simulink model "radia_optuna_teaching"  (R2026a)
settings: Solver=FixedStepDiscrete  StopTime=1.4  FixedStep=0.1
model workspace (MAT data in the model file):
  radia_optuna_teaching_exercise = "quadratic"
  radia_optuna_teaching_parameters = radia.optuna.OptimizationParameter
  radia_optuna_teaching_parameters.Name = "x"
  radia_optuna_teaching_parameters.Value = 0
  radia_optuna_teaching_parameters.Minimum = -1
  radia_optuna_teaching_parameters.Maximum = 1
settings Model: Creator=Administrator  LastModifiedBy=Administrator

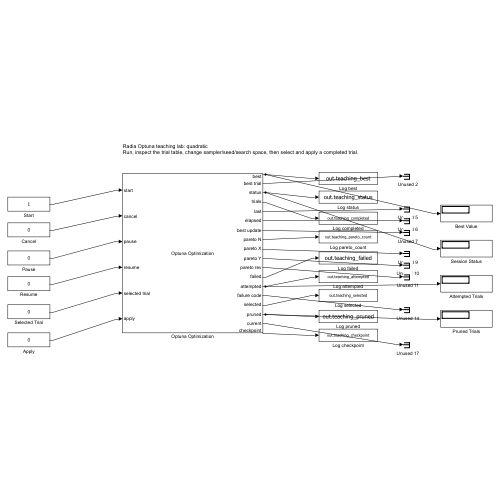
[thumbnail: Simulink's stored preview of the top-level diagram]
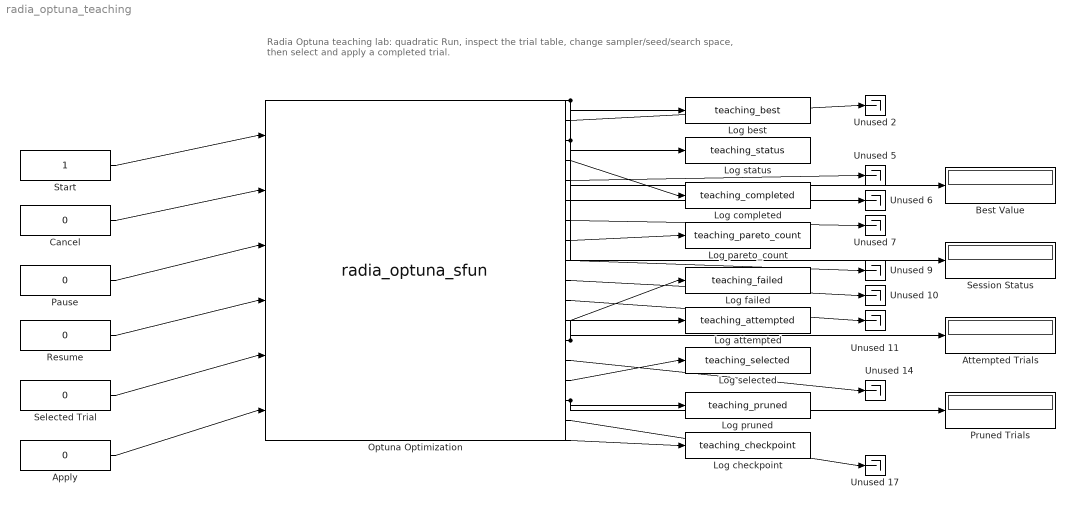
== system radia_optuna_teaching ==
  note: Radia Optuna teaching lab: quadratic
      | Run, inspect the trial table, change sampler/seed/search space, then select and apply a completed trial.
  Apply : Constant  Value=0
  Attempted Trials : Display
  Best Value : Display
  Cancel : Constant  Value=0
  Log attempted : ToWorkspace  VariableName=teaching_attempted  SampleTime=-1
  Log best : ToWorkspace  VariableName=teaching_best  SampleTime=-1
  Log checkpoint : ToWorkspace  VariableName=teaching_checkpoint  SampleTime=-1
  Log completed : ToWorkspace  VariableName=teaching_completed  SampleTime=-1
  Log failed : ToWorkspace  VariableName=teaching_failed  SampleTime=-1
  Log pareto_count : ToWorkspace  VariableName=teaching_pareto_count  SampleTime=-1
  Log pruned : ToWorkspace  VariableName=teaching_pruned  SampleTime=-1
  Log selected : ToWorkspace  VariableName=teaching_selected  SampleTime=-1
  Log status : ToWorkspace  VariableName=teaching_status  SampleTime=-1
  Optuna Optimization : M-S-Function  Description=MATLAB-native Optuna session. One trial executes per sample; completed history is checkpointed and objective failures are recorded. Status: -1 failure, 0 idle, 1 complete, 2 running, 3 cancelled, 4 paused.  FunctionName=radia_optuna_sfun  Parameters=objective_fcn,num_trials,directions,storage_path,sample_time_s,strcmp(live_visualization,'on'),struct('Name',sampler_name,'Seed',seed,'Pruner',pruner_name,'Parameters',parameter_spec,'ModelName',model_name)  mask{objective_fcn='radia.optuna.teachingQuadraticObjective', num_trials=12, directions="minimize", storage_path='C:\temp\radia_optuna_teaching_quadratic.mat', sample_time_s=0.10000000000000001, live_visualization=off, sampler_name=tpe, seed=20260829, pruner_name=median, parameter_spec=radia_optuna_teaching_parameters, model_name='radia_optuna_teaching'}
      mask prompts: objective_fcn "Objective function"; num_trials "Number of trials"; directions "Objective directions"; storage_path "Study MAT file"; sample_time_s "Trial sample time (s)"; live_visualization "External MATLAB monitor"; sampler_name "Sampler"; seed "Sampler seed ([] = fresh)"; pruner_name "Pruner"; parameter_spec "OptimizationParameter array ([] = Trial objective)"; model_name "Model to update"
      mask help: MATLAB-native Optuna session. One trial executes per sample; completed history is checkpointed and objective failures are recorded. Status: -1 failure, 0 idle, 1 complete, 2 running, 3 cancelled, 4 paused.
      mask TypeOptions sampler_name: auto | random | tpe | cmaes | motpe | nsgaii | gp | nsgaiii | bruteforce | qmc
      mask TypeOptions pruner_name: none | median | hyperband | percentile | patient | successivehalving | threshold
      mask Display: disp('Optuna Optimization');port_label('input',1,'start');port_label('input',2,'cancel');port_label('input',3,'pause');port_label('input',4,'resume');port_label('input',5,'selected trial');port_label('input',6,'apply');port_label('output',1,'best');port_label('output',2,'best trial');port_label('output',3,'status');port_label('output',4,'trials');port_label('output',5,'last');port_label('output',6,'elapsed');port_label('output',7,'best update');port_label('output',8,'pareto N');port_label('output',9,'pareto X');port_label('output',10,'pareto Y');port_label('output',11,'pareto rev');port_label('output',12,'failed');port_label('output',13,'attempted');port_label('output',14,'failure code');port_label('output',15,'selected');port_label('output',16,'pruned');port_label('output',17,'current');port_label('output',18,'checkpoint');
  Pause : Constant  Value=0
  Pruned Trials : Display
  Resume : Constant  Value=0
  Selected Trial : Constant  Value=0
  Session Status : Display
  Start : Constant
  Unused {2,5..7,9..11,14,17} (9 alike) : Terminator
  wires:
  Start/1 -> Optuna Optimization/1
  Cancel/1 -> Optuna Optimization/2
  Pause/1 -> Optuna Optimization/3
  Resume/1 -> Optuna Optimization/4
  Selected Trial/1 -> Optuna Optimization/5
  Apply/1 -> Optuna Optimization/6
  Optuna Optimization/1 -> Log best/1, Best Value/1
  Optuna Optimization/3 -> Log status/1, Session Status/1
  Optuna Optimization/4 -> Log completed/1
  Optuna Optimization/8 -> Log pareto_count/1
  Optuna Optimization/12 -> Log failed/1
  Optuna Optimization/13 -> Log attempted/1, Attempted Trials/1
  Optuna Optimization/15 -> Log selected/1
  Optuna Optimization/16 -> Log pruned/1, Pruned Trials/1
  Optuna Optimization/18 -> Log checkpoint/1
  Optuna Optimization/2 -> Unused 2/1
  Optuna Optimization/5 -> Unused 5/1
  Optuna Optimization/6 -> Unused 6/1
  Optuna Optimization/7 -> Unused 7/1
  Optuna Optimization/9 -> Unused 9/1
  Optuna Optimization/10 -> Unused 10/1
  Optuna Optimization/11 -> Unused 11/1
  Optuna Optimization/14 -> Unused 14/1
  Optuna Optimization/17 -> Unused 17/1
